simulink model "MOD_SEMPLICE"  (R2024a)
settings: Solver=VariableStepAuto  StartTime=0.0  StopTime=3000  RelTol=1e-3
values from neighbouring files (symbols this model uses):
  cp = [1e-05 1e-05 1e-05 1e-05 1e-05 1e-05 1e-05 1e-05 1e-05 1e-05 1e-05 1e-05 ... (3015 elements, 15x201)]    [CP.mat]
  pitch = [1 3 5 7 9 11 13 15 17 19 21 23 ... (15 elements, 1x15)]    [CP.mat]
  TSR = [0 0.1 0.2 0.3 0.4 0.5 0.6 0.7 0.8 0.9 1 1.1 ... (201 elements, 1x201)]    [CP.mat]
libraries: simulink x4
settings Model: Creator=emanuele  LastModifiedBy=emanuele

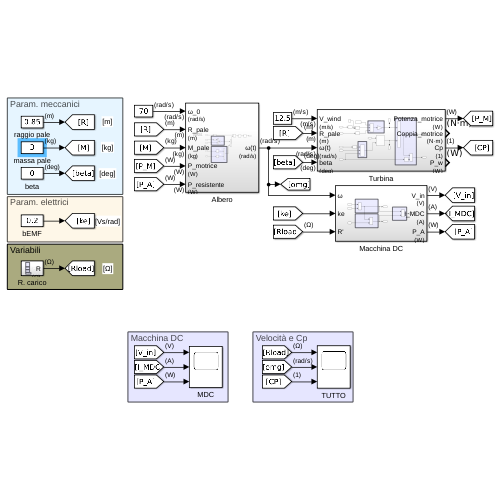
[thumbnail: Simulink's stored preview of the top-level diagram]
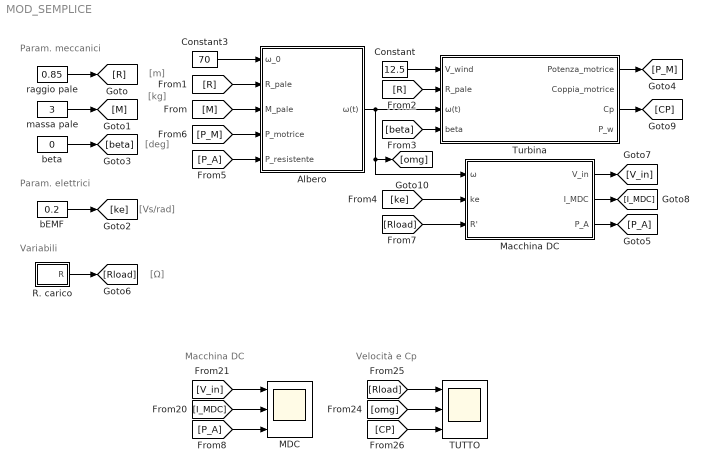
== system MOD_SEMPLICE ==
  note: Macchina DC
  note: [kg]
  note: [deg]
  note: Param. meccanici
  note: [m]
  note: Param. elettrici
  note: [Vs/rad]
  note: Variabili
  note: [Ω]
  note: Velocità e Cp
  Albero : Subsystem
  Constant : Constant  Value=12.5
  Constant3 : Constant  Value=70
  MDC : Scope  NumInputPorts=3
  Macchina DC : Subsystem
  R. carico : Subsystem
  TUTTO : Scope  NumInputPorts=3
  Turbina : Subsystem
  bEMF : Constant  Value=0.2
  beta : Constant  Value=0
  massa pale : Constant  Value=3
  raggio pale : Constant  Value=0.85
  wires:
  Constant/1 -> Turbina/1(V_wind)
  [R] -> Turbina/2(R_pale)
  [beta] -> Turbina/4(beta)
  [R] -> Albero/2(R_pale)
  [M] -> Albero/3(M_pale)
  [P_M] -> Albero/4(P_motrice)
  Constant3/1 -> Albero/1(ω_0)
  Albero/1(ω(t)) -> [omg], Macchina DC/1(ω), Turbina/3(ω(t))
  Turbina/1(Potenza_motrice) -> [P_M]
  [P_A] -> Albero/5(P_resistente)
  raggio pale/1 -> [R]
  beta/1 -> [beta]
  massa pale/1 -> [M]
  bEMF/1 -> [ke]
  [ke] -> Macchina DC/2(ke)
  Macchina DC/3(P_A) -> [P_A]
  R. carico/1(R) -> [Rload]
  [Rload] -> Macchina DC/3(R')
  Macchina DC/2(I_MDC) -> [I_MDC]
  Macchina DC/1(V_in) -> [V_in]
  [CP] -> TUTTO/3
  [omg] -> TUTTO/2
  [Rload] -> TUTTO/1
  [V_in] -> MDC/1
  [I_MDC] -> MDC/2
  [P_A] -> MDC/3
  Turbina/3(Cp) -> [CP]

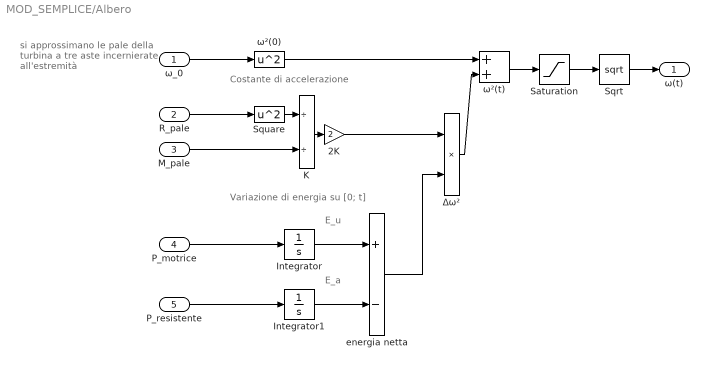
== system MOD_SEMPLICE/Albero ==
  note: E_u
  note: E_a
  note: si approssimano le pale
      | della turbina a tre aste
      | incernierate all'estremità
  note: Variazione di energia su [0; t]
  note: Costante di accelerazione
  ω_0 : Inport  Unit=rad/s
  R_pale : Inport  Port=2  Unit=m
  M_pale : Inport  Port=3  Unit=kg
  P_motrice : Inport  Port=4  Unit=W
  P_resistente : Inport  Port=5  Unit=W
  2K : Gain  Gain=2
  Integrator : Integrator
  Integrator1 : Integrator
  K : Product  Inputs=//
  Saturation : Saturate  UpperLimit=10e6  LowerLimit=0
  Sqrt : Sqrt
  Square : Math  Operator=square
  energia netta : Sum  Inputs=+-
  Δω² : Product
  ω²(0) : Math  Operator=square
  ω²(t) : Sum
  ω(t) : Outport  Unit=rad/s
  wires:
  Saturation/1 -> Sqrt/1
  Integrator1/1 -> energia netta/2
  2K/1 -> Δω²/1
  ω²(t)/1 -> Saturation/1
  ω_0/1 -> ω²(0)/1
  ω²(0)/1 -> ω²(t)/1
  P_motrice/1 -> Integrator/1
  Square/1 -> K/1
  Δω²/1 -> ω²(t)/2
  P_resistente/1 -> Integrator1/1
  R_pale/1 -> Square/1
  Integrator/1 -> energia netta/1
  energia netta/1 -> Δω²/2
  Sqrt/1 -> ω(t)/1
  K/1 -> 2K/1
  M_pale/1 -> K/2

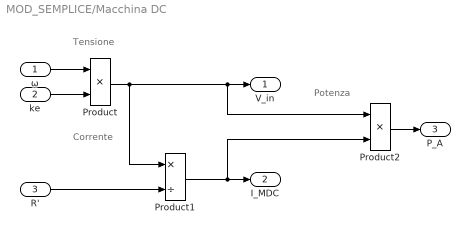
== system MOD_SEMPLICE/Macchina DC ==
  note: Tensione
  note: Corrente
  note: Potenza
  ω : Inport
  ke : Inport  Port=2
  R' : Inport  Port=3
  Product : Product
  Product1 : Product  Inputs=*/
  Product2 : Product
  V_in : Outport  Unit=V
  I_MDC : Outport  Port=2  Unit=A
  P_A : Outport  Port=3  Unit=W
  wires:
  ke/1 -> Product/2
  ω/1 -> Product/1
  R'/1 -> Product1/2
  Product1/1 -> Product2/2, I_MDC/1
  Product/1 -> Product1/1, Product2/1, V_in/1
  Product2/1 -> P_A/1

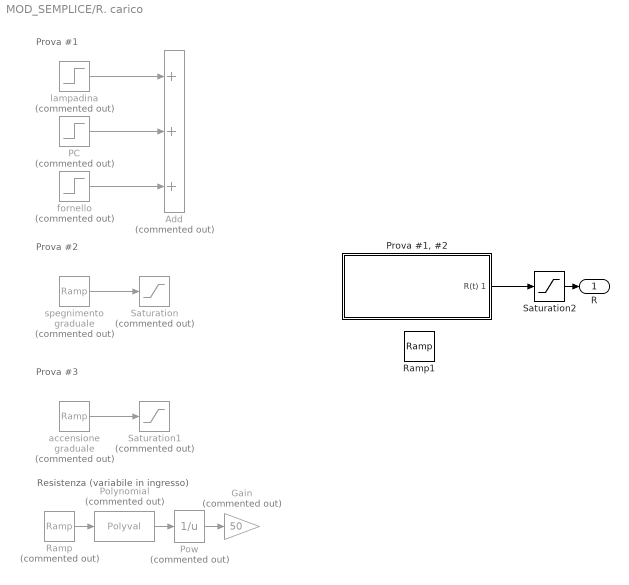
== system MOD_SEMPLICE/R. carico ==
  note: Prova #1
  note: Prova #2
  note: Prova #3
  note: Resistenza (variabile in ingresso)
  Add : Sum  Commented=on  Inputs=+++
  Gain : Gain  Commented=on  Gain=50
  PC : Step  Commented=on  Time=1200  After=90  SampleTime=0
  Polynomial : Polyval  Commented=on  Coefs=[10e-4 0 0]
  Pow : Math  Commented=on  Operator=reciprocal  SignedPower=on  RndMeth=Zero
  "Prova #1, #2" : Subsystem
  Ramp : simulink/Sources/Ramp  Commented=on  slope=0.12  start=100  InitialOutput=0.1
  Ramp1 : simulink/Sources/Ramp  slope=-4e-4  start=300  InitialOutput=1
  Saturation : Saturate  Commented=on  UpperLimit=1000  LowerLimit=0
  Saturation1 : Saturate  Commented=on  UpperLimit=200  LowerLimit=0
  Saturation2 : Saturate  UpperLimit=10e6  LowerLimit=0.15
  accensione graduale : simulink/Sources/Ramp  Commented=on  slope=2  start=900  InitialOutput=0
  fornello : Step  Commented=on  Time=1500  After=900  SampleTime=0
  lampadina : Step  Commented=on  Time=900  After=10  SampleTime=0
  spegnimento graduale : simulink/Sources/Ramp  Commented=on  slope=-10  start=900  InitialOutput=1000
  R : Outport  Unit=Ω
  wires:
  lampadina/1 -> Add/1
  PC/1 -> Add/2
  fornello/1 -> Add/3
  spegnimento graduale/1 -> Saturation/1
  accensione graduale/1 -> Saturation1/1
  Pow/1 -> Gain/1
  Ramp/1 -> Polynomial/1
  Polynomial/1 -> Pow/1
  Saturation2/1 -> R/1
  "Prova #1, #2"/1(R(t) 1) -> Saturation2/1

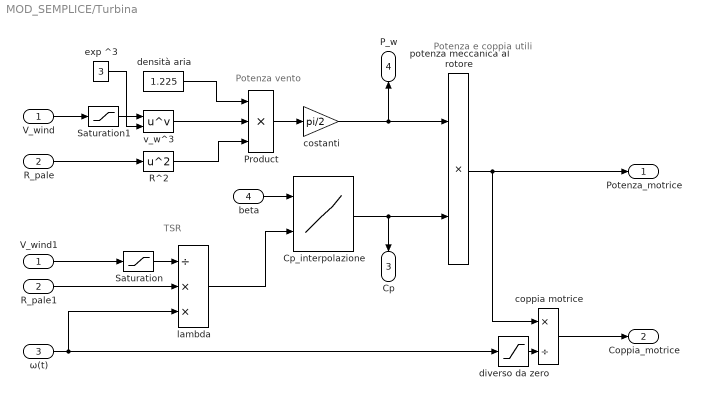
== system MOD_SEMPLICE/Turbina ==
  note: Potenza e coppia utili
  note: TSR
  note: Potenza vento
  V_wind : Inport  Unit=m/s
  R_pale : Inport  Port=2  Unit=m
  ω(t) : Inport  Port=3  Unit=rad/s
  beta : Inport  Port=4  Unit=deg
  Cp_interpolazione : Lookup_n-D  BreakpointsForDimension1=pitch  BreakpointsForDimension2=TSR  Table=cp  InterpMethod=Cubic spline  InternalRulePriority=Speed  RndMeth=Simplest
      settings: InputPortMap=u0,u1
  Product : Product  Inputs=***
  R^2 : Math  Operator=square
  R_pale1 : InportShadow  Port=2  Unit=m
  Saturation : Saturate  UpperLimit=15  LowerLimit=1
  Saturation1 : Saturate  UpperLimit=15  LowerLimit=1
  V_wind1 : InportShadow  Unit=m/s
  coppia motrice : Product  Inputs=*/
  costanti : Gain  Gain=pi/2
  densità aria : Constant  Value=1.225
  diverso da zero : Saturate  UpperLimit=10e3  LowerLimit=0.1
  exp ^3 : Constant  Value=3
  lambda : Product  Inputs=/**
  potenza meccanica al rotore : Product
  v_w^3 : Math  Operator=pow
  Potenza_motrice : Outport  Unit=W
  Coppia_motrice : Outport  Port=2  Unit=N*m
  Cp : Outport  Port=3  Unit=1
  P_w : Outport  Port=4  Unit=W
  wires:
  potenza meccanica al rotore/1 -> coppia motrice/1, Potenza_motrice/1
  R_pale/1 -> R^2/1
  V_wind/1 -> Saturation1/1
  densità aria/1 -> Product/1
  v_w^3/1 -> Product/2
  R^2/1 -> Product/3
  Product/1 -> costanti/1
  Cp_interpolazione/1 -> potenza meccanica al rotore/2, Cp/1
  beta/1 -> Cp_interpolazione/1
  lambda/1 -> Cp_interpolazione/2
  ω(t)/1 -> diverso da zero/1, lambda/3
  diverso da zero/1 -> coppia motrice/2
  coppia motrice/1 -> Coppia_motrice/1
  costanti/1 -> potenza meccanica al rotore/1, P_w/1
  exp ^3/1 -> v_w^3/2
  R_pale1/1 -> lambda/2
  V_wind1/1 -> Saturation/1
  Saturation/1 -> lambda/1
  Saturation1/1 -> v_w^3/1

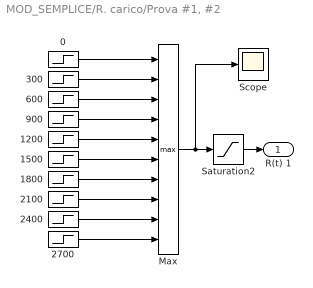
== system MOD_SEMPLICE/R. carico/Prova #1, #2 ==
  0 : Step  Time=300  Before=1.6  After=0  SampleTime=0
  1200 : Step  Time=1500  Before=0.6  After=0  SampleTime=0
  1500 : Step  Time=1800  Before=0.4  After=0  SampleTime=0
  1800 : Step  Time=2100  Before=0.4  After=0  SampleTime=0
  2100 : Step  Time=2400  Before=0.2  After=0  SampleTime=0
  2400 : Step  Time=2700  Before=0.2  After=0  SampleTime=0
  2700 : Step  Time=2700  After=1.6  SampleTime=0
  300 : Step  Time=600  Before=1.3  After=0  SampleTime=0
  600 : Step  Time=900  Before=1  After=0  SampleTime=0
  900 : Step  Time=1200  Before=0.8  After=0  SampleTime=0
  Max : MinMax  Function=max  Inputs=10
  Saturation2 : Saturate  UpperLimit=10e6  LowerLimit=0.15
  Scope : Scope
  R(t) 1 : Outport
  wires:
  2400/1 -> Max/9
  600/1 -> Max/3
  Max/1 -> Scope/1, Saturation2/1
  1800/1 -> Max/7
  2700/1 -> Max/10
  1500/1 -> Max/6
  1200/1 -> Max/5
  0/1 -> Max/1
  900/1 -> Max/4
  2100/1 -> Max/8
  300/1 -> Max/2
  Saturation2/1 -> R(t) 1/1
